simulink model "sync_mach_cont_sim_simple"  (R2017a)
settings: Solver=ode23tb  StartTime=0.0  StopTime=10.0  FixedStep=1e-5  RelTol=1e-3
undefined symbols (not defined in the file or in its folder): DiscIntNeverNeededParam
settings Model: Creator=krovchen  LastModifiedBy=krovchen
settings OptimizationCC: DefaultParameterBehavior=Inlined  UseDivisionForNetSlopeComputation=on  UseFloatMulNetSlope=on  InlineInvariantSignals=on  PassReuseOutputArgsAs=Individual arguments  ZeroExternalMemoryAtStartup=off  ZeroInternalMemoryAtStartup=off  NoFixptDivByZeroProtection=on  EfficientFloat2IntCast=on
settings DebuggingCC: ParameterTunabilityLossMsg=error
settings SFSimCC: MATLABDynamicMemAlloc=off
settings RTWCC: SystemTargetFile=ert.tlc  GenCodeOnly=on  GenerateMakefile=off  PackageGeneratedCodeAndArtifacts=on  PackageName=v1_model_export  TemplateMakefile=RTW.MSVCBuild  Description=Create Visual C/C++ Solution File for Embedded Coder  GenerateReport=on  IncludeHyperlinkInReport=on  LaunchReport=on  TargetLang=C++  GenerateTraceInfo=on  GenerateTraceReport=on  GenerateTraceReportSl=on  GenerateTraceReportSf=on  GenerateTraceReportEml=on
settings CodeAppCC: ForceParamTrailComments=on  IgnoreCustomStorageClasses=off  OperatorAnnotations=on  SimulinkDataObjDesc=on  SFDataObjDesc=on  MATLABFcnDesc=on  CustomSymbolStrGlobalVar=rt$N$M  CustomSymbolStrType=$N$M  CustomSymbolStrFcn=$N$M$F  CustomSymbolStrMacro=$N$M  InsertBlockDesc=on  MATLABSourceComments=on
settings ERTTargetCC: TargetLangStandard=C++03 (ISO)  GenerateSampleERTMain=on  MultiInstanceERTCode=on  CodeInterfacePackaging=C++ class  SupportContinuousTime=on  InlinedParameterPlacement=NonHierarchical  RootIOFormat=Structure reference  ERTCustomFileTemplate=example_file_process.tlc

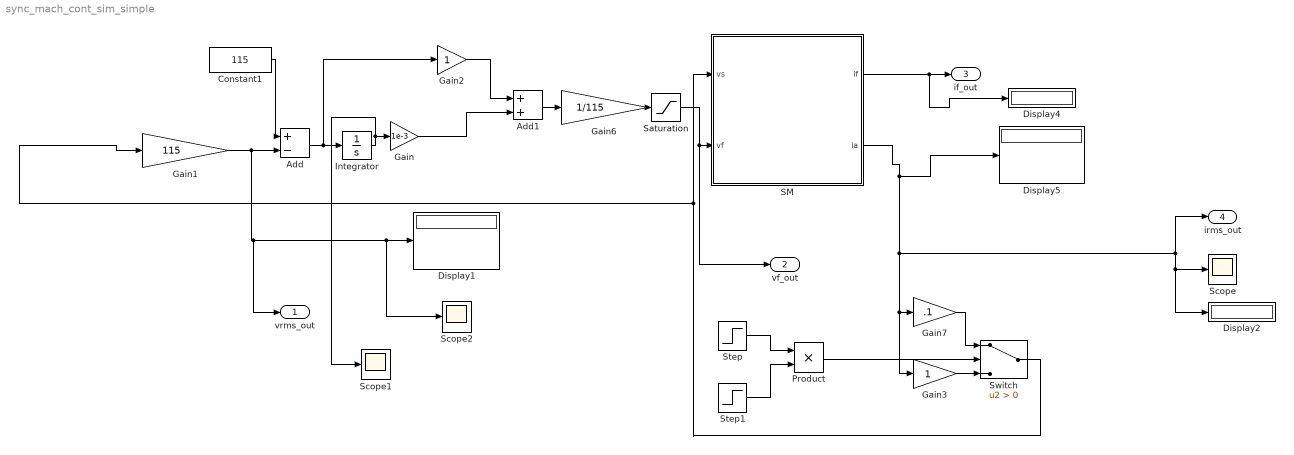
== system sync_mach_cont_sim_simple ==
  Add : Sum  Inputs=+-
  Add1 : Sum
  Constant1 : Constant  Value=115
  Display{1..2,4..5} (4 alike) : Display
  Gain : Gain  Gain=1e-3
  Gain1 : Gain  Gain=115
  Gain2 : Gain
  Gain3 : Gain
  Gain6 : Gain  Gain=1/115
  Gain7 : Gain  Gain=.1
  Integrator : Integrator  LimitOutput=on  UpperSaturationLimit=1  LowerSaturationLimit=-1
  Product : Product
  SM : Subsystem
      mask Display:
      | plot(-1.5,-1.5,1.5,1.5,cos(0:.01:7),sin(0:.01:7),[-.5 -1 1 .5],[-.866 -1.2 -1.2 -.866] )
      | disp('SYNCHRONOUS\nMACHINE')
  Saturation : Saturate  UpperLimit=1  LowerLimit=-1
  Scope : Scope
  Scope1 : Scope
  Scope2 : Scope
  Step : Step  Time=5  SampleTime=0
  Step1 : Step  Time=7  Before=1  After=0  SampleTime=0
  Switch : Switch  Criteria=u2 > Threshold
  vrms_out : Outport
  vf_out : Outport  Port=2
  if_out : Outport  Port=3
  irms_out : Outport  Port=4
  wires:
  Add1/1 -> Gain6/1
  Gain6/1 -> Saturation/1
  Switch/1 -> Gain1/1, SM/1(vs)
  Gain1/1 -> vrms_out/1, Scope2/1, Display1/1, Add/2
  Constant1/1 -> Add/1
  Add/1 -> Gain2/1, Integrator/1
  Integrator/1 -> Scope1/1, Gain/1
  Gain/1 -> Add1/2
  Gain2/1 -> Add1/1
  SM/2(ia) -> Display5/1, Display2/1, Scope/1, irms_out/1, Gain3/1, Gain7/1
  Step/1 -> Product/1
  Step1/1 -> Product/2
  Product/1 -> Switch/2
  Gain7/1 -> Switch/1
  Gain3/1 -> Switch/3
  Saturation/1 -> vf_out/1, SM/2(vf)
  SM/1(if) -> Display4/1, if_out/1

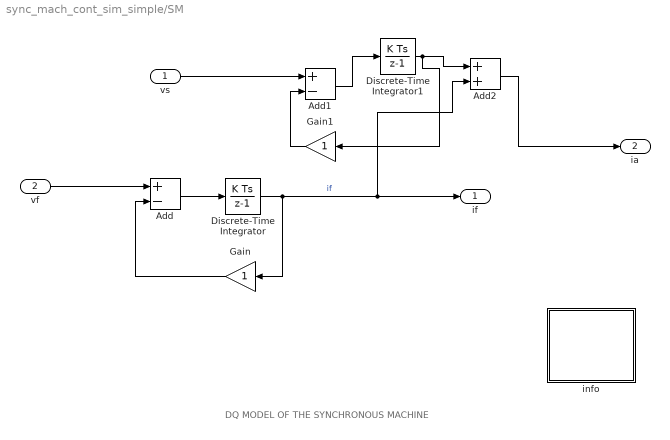
== system sync_mach_cont_sim_simple/SM ==
  note: DQ MODEL OF THE SYNCHRONOUS MACHINE
  vs : Inport
  vf : Inport  Port=2
  Add : Sum  Inputs=+-
  Add1 : Sum  Inputs=+-
  Add2 : Sum
  Discrete-Time Integrator : DiscreteIntegrator  InitialConditionSetting=State (most efficient)  SampleTime=-1  ICPrevOutput=DiscIntNeverNeededParam  ICPrevScaledInput=DiscIntNeverNeededParam
  Discrete-Time Integrator1 : DiscreteIntegrator  InitialConditionSetting=State (most efficient)  SampleTime=-1  ICPrevOutput=DiscIntNeverNeededParam  ICPrevScaledInput=DiscIntNeverNeededParam
  Gain : Gain
  Gain1 : Gain
  info : Subsystem
      settings: OpenFcn=helpview(which('smeq0.htm'));
      mask Display:
      | plot(-1.5,-1.5,1.5,1.5,cos(0:.01:7),sin(0:.01:7) )
      | disp('Equations')
  if : Outport
  ia : Outport  Port=2
  wires:
  vs/1 -> Add1/1
  vf/1 -> Add/1
  Discrete-Time Integrator/1 -> Gain/1, Add2/2, if/1  "if"
  Add2/1 -> ia/1
  Gain/1 -> Add/2
  Add/1 -> Discrete-Time Integrator/1
  Add1/1 -> Discrete-Time Integrator1/1
  Discrete-Time Integrator1/1 -> Gain1/1, Add2/1
  Gain1/1 -> Add1/2

== system sync_mach_cont_sim_simple/SM/info ==
  note: This  demonstration  illustrates  the dynamics of a synchronous generator, initially
      | at no load,  following a three-phase short circuit at the terminals.
  note: Synchronous machine transients
      | under shortcircuit
